simulink model "cic_bitwidths"  (Simulink 6.6)
settings: Solver=VariableStepDiscrete  SolverMode=SingleTasking  StartTime=0.0  StopTime=4096/10e6  RelTol=1e-3
libraries: xbsIndex_r4 x48
settings Model: Creator=lcrockett  LastModifiedBy=lcrockett
settings DataIOCC: SignalLoggingName=sigsOut
settings OptimizationCC: InlineParams=on  InlineInvariantSignals=on
settings DebuggingCC: SignalResolutionControl=TryResolveAllWithWarning  SolverPrmCheckMsg=none  MultiTaskDSMMsg=warning  MultiTaskCondExecSysMsg=none  StrictBusMsg=None
settings HardwareCC: TargetUnknown=on
settings RTWCC: IncludeERTFirstTime=on
settings GRTTargetCC: ModelReferenceCompliant=off  MatFileLogging=off

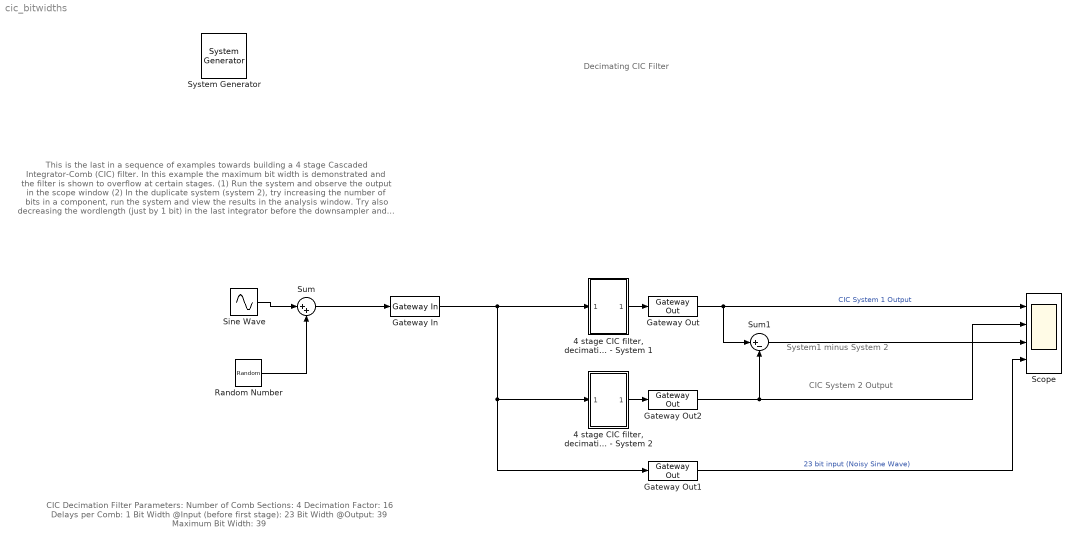
== system cic_bitwidths ==
  note: This is the last in a sequence of examples towards building a 4 stage Cascaded Integrator-Comb (CIC) filter.
      | In this example the maximum bit width is demonstrated and the filter is shown to overflow at certain stages.
      |
      | (1) Run the system and observe the output in the scope window
      |
      | (2) In the duplicate system (system 2), try increasing the number of bits in a component, run the system and view the results in the analysis window.
      | Try also decreasing the wordlength (just by 1 bit) in the last integrator before the downsampler and view the difference between the two signals in the scope window.
      | Observe the results in the scope window for different wordlengths at different points in the filter cascade.
  note: Decimating CIC Filter
  note: CIC Decimation Filter Parameters:
      | Number of Comb Sections: 4
      | Decimation Factor: 16
      | Delays per Comb: 1
      | Bit Width @Input (before first stage): 23
      | Bit Width @Output: 39
      | Maximum Bit Width: 39
  note: CIC System 2 Output
  note: System1 minus System 2
  " System Generator" : xbsIndex_r4/ System Generator  Tag=genX  SystemSampleTime=-1  xilinxfamily=virtex2p  part=xc2vp30  speed=-7  package=ff896  synthesis_tool=XST  clock_wrapper=Clock Enables  directory=./netlist  testbench=off  simulink_period=1/10e6  sysclk_period=10  dcm_input_clock_period=100  incr_netlist=off  trim_vbits=Everywhere in SubSystem  dbl_ovrd=No Where in SubSystem  core_generation=According to Block Masks  run_coregen=off  deprecated_control=off  eval_field=0  block_type=sysgen
      settings: block_version=8.2
  "4 stage CIC filter, decimation by 16 - System 1" : Subsystem
  "4 stage CIC filter, decimation by 16 - System 2" : Subsystem
  Gateway In : xbsIndex_r4/Gateway In  arith_type="Signed  (2's comp)"  n_bits=23  bin_pt=0  quantization=Truncate  overflow=Flag as error  period=1/10e6  dbl_ovrd=off  timing_constraint=None  locs_specified=off  LOCs={}  block_type=gatewayin
      settings: infoedit="Gateway in block.  Converts inputs of type Simulink integer, double and fixed point to  Xilinx fixed point type.<P><P>Hardware notes:  In hardware these blocks become top level input ports."  xl_area=[0, 0, 0, 0, 0, 0, 0]  block_version=VER_STRING_GOES_HERE
  Gateway Out : xbsIndex_r4/Gateway Out  hdl_port=on  timing_constraint=None  locs_specified=off  LOCs={}  block_type=gatewayout
      settings: infoedit="Gateway out block.  Converts Xilinx fixed point inputs into ouputs of type Simulink integer, double, or fixed point.<P><P>Hardware notes:  In hardware these blocks become top level output ports or are discarded, depending on how they are configured."  xl_area=[0, 0, 0, 0, 0, 0, 0]  block_version=VER_STRING_GOES_HERE
  Gateway Out1 : xbsIndex_r4/Gateway Out  hdl_port=on  timing_constraint=None  locs_specified=off  LOCs={}  block_type=gatewayout
      settings: infoedit="Gateway out block.  Converts Xilinx fixed point inputs into ouputs of type Simulink integer, double, or fixed point.<P><P>Hardware notes:  In hardware these blocks become top level output ports or are discarded, depending on how they are configured."  xl_area=[0, 0, 0, 0, 0, 0, 0]  block_version=VER_STRING_GOES_HERE
  Gateway Out2 : xbsIndex_r4/Gateway Out  hdl_port=on  timing_constraint=None  locs_specified=off  LOCs={}  block_type=gatewayout
      settings: infoedit="Gateway out block.  Converts Xilinx fixed point inputs into ouputs of type Simulink integer, double, or fixed point.<P><P>Hardware notes:  In hardware these blocks become top level output ports or are discarded, depending on how they are configured."  xl_area=[0, 0, 0, 0, 0, 0, 0]  block_version=VER_STRING_GOES_HERE
  Random Number : RandomNumber  Variance=393.216e+8  SampleTime=0
  Scope : Scope  NumInputPorts=4
      settings: TimeRange=0.00045  YMin=-1e+011~-1e+011~-1~-4e+006  YMax=1e+011~1e+011~1~4e+006
  Sine Wave : Sin  Amplitude=1.39810133333333e+6  Frequency=20000*2*pi  SampleTime=0
  Sum : Sum  Inputs=|++  SaturateOnIntegerOverflow=on
  Sum1 : Sum  Inputs=|+-  SaturateOnIntegerOverflow=on
  wires:
  Gateway In/1 -> "4 stage CIC filter, decimation by 16 - System 1"/1(In1), Gateway Out1/1, "4 stage CIC filter, decimation by 16 - System 2"/1(In1)
  "4 stage CIC filter, decimation by 16 - System 1"/1(Out1) -> Gateway Out/1
  Gateway Out/1 -> Scope/1, Sum1/1  "CIC System 1 Output"
  Sine Wave/1 -> Sum/1
  Random Number/1 -> Sum/2
  Sum/1 -> Gateway In/1
  "4 stage CIC filter, decimation by 16 - System 2"/1(Out1) -> Gateway Out2/1
  Gateway Out2/1 -> Scope/2, Sum1/2
  Gateway Out1/1 -> Scope/4  "23 bit input (Noisy Sine Wave)"
  Sum1/1 -> Scope/3

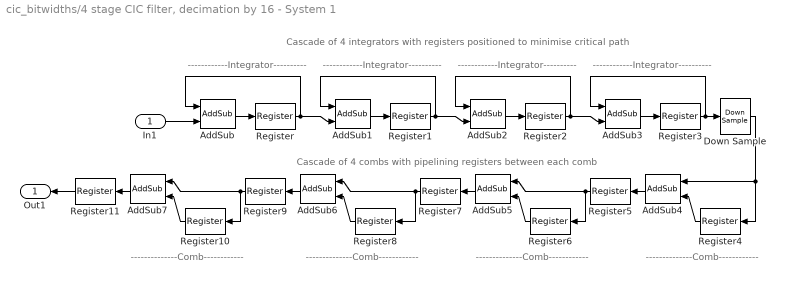
== system cic_bitwidths/4 stage CIC filter, decimation by 16 - System 1 ==
  note: ------------Integrator----------
  note: ------------Integrator----------
  note: ------------Integrator----------
  note: ------------Integrator----------
  note: --------------Comb------------
  note: --------------Comb------------
  note: --------------Comb------------
  note: --------------Comb------------
  note: Cascade of 4 integrators with registers positioned to minimise critical path
  note: Cascade of 4 combs with pipelining registers between each comb
  In1 : Inport
  AddSub{,1..3} (4 alike) : xbsIndex_r4/AddSub  mode=Addition  use_carryin=off  use_carryout=off  en=off  latency=0  precision=User Defined  arith_type="Signed  (2's comp)"  n_bits=39  bin_pt=0  quantization=Truncate  overflow=Wrap  dbl_ovrd=off  use_behavioral_HDL=on  pipelined=off  use_rpm=on  block_type=addsub
      settings: xl_area=[0, 0, 0, 0, 0, 0, 0]  block_version=VER_STRING_GOES_HERE
  AddSub{4..7} (4 alike) : xbsIndex_r4/AddSub  Orientation=left  mode=Subtraction  use_carryin=off  use_carryout=off  en=off  latency=0  precision=User Defined  arith_type="Signed  (2's comp)"  n_bits=39  bin_pt=0  quantization=Truncate  overflow=Wrap  dbl_ovrd=off  use_behavioral_HDL=on  pipelined=off  use_rpm=on  block_type=addsub
      settings: xl_area=[0, 0, 0, 0, 0, 0, 0]  block_version=VER_STRING_GOES_HERE
  Down Sample : xbsIndex_r4/Down Sample  sample_ratio=16  sample_phase="Last Value of Frame  (most efficient)"  en=off  latency=1  dbl_ovrd=off  block_type=dsamp
      settings: xl_area=[0, 0, 0, 0, 0, 0, 0]  block_version=VER_STRING_GOES_HERE
  Register{,1..3} (4 alike) : xbsIndex_r4/Register  init=0  rst=off  en=off  dbl_ovrd=off  block_type=register
      settings: xl_area=[0, 0, 0, 0, 0, 0, 0]  block_version=VER_STRING_GOES_HERE
  Register{4..11} (8 alike) : xbsIndex_r4/Register  Orientation=left  init=0  rst=off  en=off  dbl_ovrd=off  block_type=register
      settings: xl_area=[0, 0, 0, 0, 0, 0, 0]  block_version=VER_STRING_GOES_HERE
  Out1 : Outport  Orientation=left
  wires:
  AddSub/1 -> Register/1
  Register/1 -> AddSub/1, AddSub1/2
  AddSub1/1 -> Register1/1
  Register1/1 -> AddSub1/1, AddSub2/2
  AddSub2/1 -> Register2/1
  Register2/1 -> AddSub2/1, AddSub3/2
  AddSub3/1 -> Register3/1
  Register3/1 -> AddSub3/1, Down Sample/1
  Down Sample/1 -> AddSub4/1, Register4/1
  Register4/1 -> AddSub4/2
  AddSub4/1 -> Register5/1
  Register5/1 -> AddSub5/1, Register6/1
  Register6/1 -> AddSub5/2
  AddSub5/1 -> Register7/1
  Register7/1 -> AddSub6/1, Register8/1
  Register8/1 -> AddSub6/2
  AddSub6/1 -> Register9/1
  Register9/1 -> AddSub7/1, Register10/1
  Register10/1 -> AddSub7/2
  AddSub7/1 -> Register11/1
  In1/1 -> AddSub/2
  Register11/1 -> Out1/1

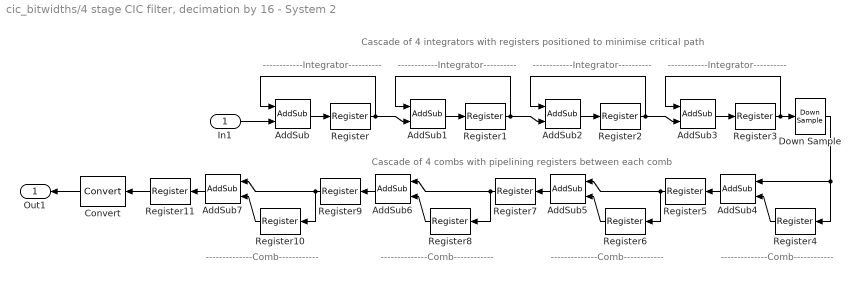
== system cic_bitwidths/4 stage CIC filter, decimation by 16 - System 2 ==
  note: ------------Integrator----------
  note: ------------Integrator----------
  note: ------------Integrator----------
  note: ------------Integrator----------
  note: --------------Comb------------
  note: --------------Comb------------
  note: --------------Comb------------
  note: --------------Comb------------
  note: Cascade of 4 integrators with registers positioned to minimise critical path
  note: Cascade of 4 combs with pipelining registers between each comb
  In1 : Inport
  AddSub{,1..3} (4 alike) : xbsIndex_r4/AddSub  mode=Addition  use_carryin=off  use_carryout=off  en=off  latency=0  precision=User Defined  arith_type="Signed  (2's comp)"  n_bits=39  bin_pt=0  quantization=Truncate  overflow=Wrap  dbl_ovrd=off  use_behavioral_HDL=on  pipelined=off  use_rpm=on  block_type=addsub
      settings: xl_area=[0, 0, 0, 0, 0, 0, 0]  block_version=VER_STRING_GOES_HERE
  AddSub4 : xbsIndex_r4/AddSub  Orientation=left  mode=Subtraction  use_carryin=off  use_carryout=off  en=off  latency=0  precision=User Defined  arith_type="Signed  (2's comp)"  n_bits=39  bin_pt=0  quantization=Truncate  overflow=Wrap  dbl_ovrd=off  use_behavioral_HDL=on  pipelined=off  use_rpm=on  block_type=addsub
      settings: xl_area=[0, 0, 0, 0, 0, 0, 0]  block_version=VER_STRING_GOES_HERE
  AddSub5 : xbsIndex_r4/AddSub  Orientation=left  mode=Subtraction  use_carryin=off  use_carryout=off  en=off  latency=0  precision=User Defined  arith_type="Signed  (2's comp)"  n_bits=39  bin_pt=0  quantization=Truncate  overflow=Wrap  dbl_ovrd=off  use_behavioral_HDL=on  pipelined=off  use_rpm=on  block_type=addsub
      settings: xl_area=[0, 0, 0, 0, 0, 0, 0]  block_version=VER_STRING_GOES_HERE
  AddSub6 : xbsIndex_r4/AddSub  Orientation=left  mode=Subtraction  use_carryin=off  use_carryout=off  en=off  latency=0  precision=User Defined  arith_type="Signed  (2's comp)"  n_bits=39  bin_pt=0  quantization=Truncate  overflow=Wrap  dbl_ovrd=off  use_behavioral_HDL=on  pipelined=off  use_rpm=on  block_type=addsub
      settings: xl_area=[0, 0, 0, 0, 0, 0, 0]  block_version=VER_STRING_GOES_HERE
  AddSub7 : xbsIndex_r4/AddSub  Orientation=left  mode=Subtraction  use_carryin=off  use_carryout=off  en=off  latency=0  precision=User Defined  arith_type="Signed  (2's comp)"  n_bits=50  bin_pt=0  quantization=Truncate  overflow=Wrap  dbl_ovrd=off  use_behavioral_HDL=on  pipelined=off  use_rpm=on  block_type=addsub
      settings: xl_area=[0, 0, 0, 0, 0, 0, 0]  block_version=VER_STRING_GOES_HERE
  Convert : xbsIndex_r4/Convert  Orientation=left  arith_type="Signed  (2's comp)"  n_bits=39  bin_pt=0  quantization=Truncate  overflow=Wrap  latency=0  dbl_ovrd=off  pipeline=off  block_type=convert
      settings: block_version=10.1.2
  Down Sample : xbsIndex_r4/Down Sample  sample_ratio=16  sample_phase="Last Value of Frame  (most efficient)"  en=off  latency=1  dbl_ovrd=off  block_type=dsamp
      settings: xl_area=[0, 0, 0, 0, 0, 0, 0]  block_version=VER_STRING_GOES_HERE
  Register{,1..3} (4 alike) : xbsIndex_r4/Register  init=0  rst=off  en=off  dbl_ovrd=off  block_type=register
      settings: xl_area=[0, 0, 0, 0, 0, 0, 0]  block_version=VER_STRING_GOES_HERE
  Register{4..11} (8 alike) : xbsIndex_r4/Register  Orientation=left  init=0  rst=off  en=off  dbl_ovrd=off  block_type=register
      settings: xl_area=[0, 0, 0, 0, 0, 0, 0]  block_version=VER_STRING_GOES_HERE
  Out1 : Outport  Orientation=left
  wires:
  AddSub/1 -> Register/1
  Register/1 -> AddSub/1, AddSub1/2
  AddSub1/1 -> Register1/1
  Register1/1 -> AddSub1/1, AddSub2/2
  AddSub2/1 -> Register2/1
  Register2/1 -> AddSub2/1, AddSub3/2
  AddSub3/1 -> Register3/1
  Register3/1 -> AddSub3/1, Down Sample/1
  Down Sample/1 -> AddSub4/1, Register4/1
  Register4/1 -> AddSub4/2
  AddSub4/1 -> Register5/1
  Register5/1 -> AddSub5/1, Register6/1
  Register6/1 -> AddSub5/2
  AddSub5/1 -> Register7/1
  Register7/1 -> AddSub6/1, Register8/1
  Register8/1 -> AddSub6/2
  AddSub6/1 -> Register9/1
  Register9/1 -> AddSub7/1, Register10/1
  Register10/1 -> AddSub7/2
  AddSub7/1 -> Register11/1
  In1/1 -> AddSub/2
  Register11/1 -> Convert/1
  Convert/1 -> Out1/1
